simulink model "ForceFilter2Axis"  (R2022b)
settings: configuration reference "WheelSimConfiguration" (kept outside this file)
undefined symbols (not defined in the file): simulator
libraries: simulink_extras x2
settings Model: Creator=At  LastModifiedBy=MOSA
settings ConfigSetRef: SourceName=WheelSimConfiguration  SourceLocation=Base Workspace

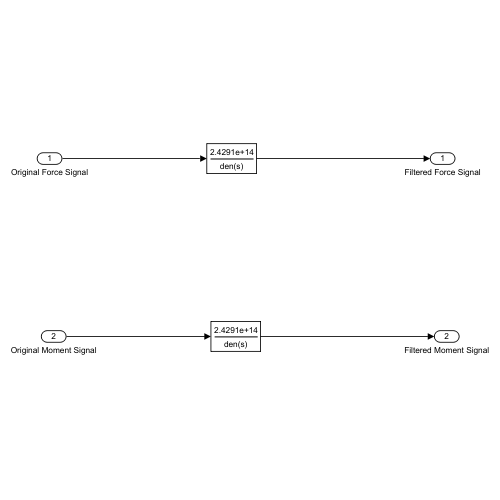
[thumbnail: Simulink's stored preview of the top-level diagram]
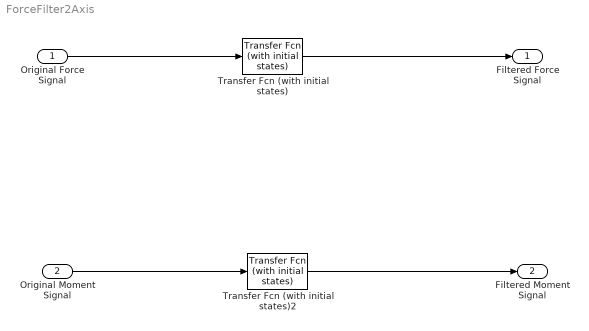
== system ForceFilter2Axis ==
  Original Force Signal : Inport
  Original Moment Signal : Inport  Port=2
  Transfer Fcn (with initial states) : simulink_extras/Additional Linear/Transfer Fcn (with initial states)  N=simulator.Forcefilter.num  D=simulator.Forcefilter.den  X0=0
  Transfer Fcn (with initial states)2 : simulink_extras/Additional Linear/Transfer Fcn (with initial states)  N=simulator.Forcefilter.num  D=simulator.Forcefilter.den  X0=0
  Filtered Force Signal : Outport
  Filtered Moment Signal : Outport  Port=2
  wires:
  Transfer Fcn (with initial states)/1 -> Filtered Force Signal/1
  Original Force Signal/1 -> Transfer Fcn (with initial states)/1
  Transfer Fcn (with initial states)2/1 -> Filtered Moment Signal/1
  Original Moment Signal/1 -> Transfer Fcn (with initial states)2/1
